simulink model "Modele_LQR_6DOF"  (R2024b)
settings: Solver=VariableStepAuto  StartTime=0.0  StopTime=50  FixedStep=0.0001  RelTol=1e-3
InitFcn:
  |     du0 = 0;
  |     du1 = 0;
  |     du2 = 0;
  |     du3 = 0;
  |     du4 = 0;
  |     du5 = 0;
  |     du6 = 0;
  |     du7 = 0;
values from neighbouring files (symbols this model uses):
  A_num = [0 0 0 0 0 0 0 0 0 0 0 0 ... (144 elements, 12x12)]    [Matrice_A_lineaire.mat]    (also in calcul_matrice_A_lineaire.m = double(A_num); resultats_stabilite.mat; testFinale.m = A_fcn(0, 0, 0, val_rll, val_ptc, val_yw, val_u, val_v, val_w; test_calcalV2.m = double(A_num))
  B = df_dcontrol    [Generate_PyMatrix.m]    (also in Parameters.m = -234.459; instabiliter_graphique.m = out.B_s.signals.values)
  Fx1 = -0.7071*force    (= -14.142)    [Parameters.m]
  Fx2 = -0.7071*force    (= -14.142)    [Parameters.m]
  Fx3 = 0    [Parameters.m]
  Fx4 = 0    [Parameters.m]
  Fx5 = 0    [Parameters.m]
  Fx6 = 0    [Parameters.m]
  Fx7 = 0.7071*force    (= 14.142)    [Parameters.m]
  Fx8 = 0.7071*force    (= 14.142)    [Parameters.m]
  Fy1 = 0.7071*force    (= 14.142)    [Parameters.m]
  Fy2 = -0.7071*force    (= -14.142)    [Parameters.m]
  Fy3 = 0    [Parameters.m]
  Fy4 = 0    [Parameters.m]
  Fy5 = 0    [Parameters.m]
  Fy6 = 0    [Parameters.m]
  Fy7 = 0.7071*force    (= 14.142)    [Parameters.m]
  Fy8 = -0.7071*force    (= -14.142)    [Parameters.m]
  Fz1 = 0    [Parameters.m]
  Fz2 = 0    [Parameters.m]
  Fz3 = -1*force    (= -20)    [Parameters.m]
  Fz4 = -1*force    (= -20)    [Parameters.m]
  Fz5 = -1*force    (= -20)    [Parameters.m]
  Fz6 = -1*force    (= -20)    [Parameters.m]
  Fz7 = 0    [Parameters.m]
  Fz8 = 0    [Parameters.m]
  I_x = 0.578    [Parameters.m]
  I_y = 0.645    [Parameters.m]
  I_z = 0.9366    [Parameters.m]
  lx1 = I_un_moteur(1)    [Calcul_Inertie_Nouveau.m]    (also in Parameters.m = 0.0194)
  lx2 = I_un_moteur(1)    [Calcul_Inertie_Nouveau.m]    (also in Parameters.m = 0.0194)
  lx3 = I_un_moteur(1)    [Calcul_Inertie_Nouveau.m]    (also in Parameters.m = -0.0317)
  lx4 = I_un_moteur(1)    [Calcul_Inertie_Nouveau.m]    (also in Parameters.m = -0.0317)
  lx5 = I_un_moteur(1)    [Calcul_Inertie_Nouveau.m]    (also in Parameters.m = 0.0317)
  lx6 = I_un_moteur(1)    [Calcul_Inertie_Nouveau.m]    (also in Parameters.m = 0.0317)
  lx7 = I_un_moteur(1)    [Calcul_Inertie_Nouveau.m]    (also in Parameters.m = -0.0194)
  lx8 = I_un_moteur(1)    [Calcul_Inertie_Nouveau.m]    (also in Parameters.m = -0.0194)
  ly1 = %.4f    [Calcul_Inertie_Nouveau.m]    (also in Parameters.m = 0.0381)
  ly2 = %.4f    [Calcul_Inertie_Nouveau.m]    (also in Parameters.m = -0.0381)
  ly3 = %.4f    [Calcul_Inertie_Nouveau.m]    (also in Parameters.m = 0.0049)
  ly4 = %.4f    [Calcul_Inertie_Nouveau.m]    (also in Parameters.m = -0.0049)
  ly5 = %.4f    [Calcul_Inertie_Nouveau.m]    (also in Parameters.m = 0.0049)
  ly6 = %.4f    [Calcul_Inertie_Nouveau.m]    (also in Parameters.m = -0.0049)
  ly7 = %.4f    [Calcul_Inertie_Nouveau.m]    (also in Parameters.m = 0.0381)
  ly8 = %.4f    [Calcul_Inertie_Nouveau.m]    (also in Parameters.m = -0.0381)
  lz1 = %.4f;\n', lx1, ly1, lz1)    [Calcul_Inertie_Nouveau.m]    (also in Parameters.m = 0.0575)
  lz2 = %.4f;\n', lx2, ly2, lz2)    [Calcul_Inertie_Nouveau.m]    (also in Parameters.m = 0.0575)
  lz3 = %.4f;\n', lx3, ly3, lz3)    [Calcul_Inertie_Nouveau.m]    (also in Parameters.m = 0.0366)
  lz4 = %.4f;\n', lx4, ly4, lz4)    [Calcul_Inertie_Nouveau.m]    (also in Parameters.m = 0.0366)
  lz5 = %.4f;\n', lx5, ly5, lz5)    [Calcul_Inertie_Nouveau.m]    (also in Parameters.m = 0.0366)
  lz6 = %.4f;\n', lx6, ly6, lz6)    [Calcul_Inertie_Nouveau.m]    (also in Parameters.m = 0.0366)
  lz7 = %.4f;\n', lx7, ly7, lz7)    [Calcul_Inertie_Nouveau.m]    (also in Parameters.m = 0.0575)
  lz8 = %.4f;\n', lx8, ly8, lz8)    [Calcul_Inertie_Nouveau.m]    (also in Parameters.m = 0.0575)
  m = 23.9    [Parameters.m]
  Q_envoyer = Q_final(:,:,1)    [Parameters.m]
  W = mass*gravity    (= 234.459)    [Generate_PyMatrix.m]    (also in Parameters.m; calcul_damping.m)
  x_rb = 0    [Parameters.m]
  x_rg = 0    [Parameters.m]
  y_rb = 0    [Parameters.m]
  y_rg = 0    [Parameters.m]
  z_rb = 0    [Parameters.m]
  z_rg = 0    [Parameters.m]
undefined symbols (not defined in the file or in its folder): sigbuilder_block
libraries: simulink x12, sharedtransform x1, dspinverses x1, SignalEditorBlockLib x1
(part 3 of 4)

== matlab function Modele_LQR_6DOF/Controller/MATLAB Function ==
  settings: updateMethod=DISCRETE
  data: R output; Q output; A output; B output; state input; Q_files input; Tau input; A_lineraire input

function [R,Q,A,B]= ABmatrix(state, Q_files, Tau, A_lineraire)
tic
    
    roll_ = state(4);
    pitch_ = state(5);
    yaw_ = state(6);
    u = state(7); %
    v = state(8); %
    w = state(9); %
    p = state(10);
    q = state(11);
    r = state(12);

    du0 = Tau(1);
    du1 = Tau(2);
    du2 = Tau(3);
    du3 = Tau(4);
    du4 = Tau(5);
    du5 = Tau(6);
    du6 = Tau(7);
    du7 = Tau(8);
    thrust = 0.1;
    importance = 0;

    % Q = Q_files;
    Q = diag([Q_files(1,1) Q_files(2,2) Q_files(3,3) Q_files(4,4) Q_files(5,5) Q_files(6,6) Q_files(7,7) Q_files(8,8) Q_files(9,9) Q_files(10,10) Q_files(11,11) Q_files(12,12)]);
    % Q = diag([80, 80, 80, 100, 100, 100, 50, 50, 50, 20, 20, 20]); % test répétition
    % Q = diag([4, 4, 4, 2, 2, 2, 1, 1, 1, 1, 1, 1]); % test ancien
    % R = diag([thrust, thrust, thrust-importance, thrust-importance, thrust-importance, thrust-importance, thrust, thrust]); 
    R = thrust*eye(8);

    radius = 0.26;
    
 % A = A_lineraire;

 % utiliser
%     A = [[0, 0, 0,   v*(sin(roll_)*sin(yaw_) + cos(roll_)*cos(yaw_)*sin(pitch_)) + w*(cos(roll_)*sin(yaw_) - cos(yaw_)*sin(pitch_)*sin(roll_)), w*cos(pitch_)*cos(roll_)*cos(yaw_) - u*cos(yaw_)*sin(pitch_) + v*cos(pitch_)*cos(yaw_)*sin(roll_), w*(cos(yaw_)*sin(roll_) - cos(roll_)*sin(pitch_)*sin(yaw_)) - v*(cos(roll_)*cos(yaw_) + sin(pitch_)*sin(roll_)*sin(yaw_)) - u*cos(pitch_)*sin(yaw_), cos(pitch_)*cos(yaw_), cos(yaw_)*sin(pitch_)*sin(roll_) - cos(roll_)*sin(yaw_), sin(roll_)*sin(yaw_) + cos(roll_)*cos(yaw_)*sin(pitch_),             0,                      0,                      0]
% [0, 0, 0, - v*(cos(yaw_)*sin(roll_) - cos(roll_)*sin(pitch_)*sin(yaw_)) - w*(cos(roll_)*cos(yaw_) + sin(pitch_)*sin(roll_)*sin(yaw_)), w*cos(pitch_)*cos(roll_)*sin(yaw_) - u*sin(pitch_)*sin(yaw_) + v*cos(pitch_)*sin(roll_)*sin(yaw_), w*(sin(roll_)*sin(yaw_) + cos(roll_)*cos(yaw_)*sin(pitch_)) - v*(cos(roll_)*sin(yaw_) - cos(yaw_)*sin(pitch_)*sin(roll_)) + u*cos(pitch_)*cos(yaw_), cos(pitch_)*sin(yaw_), cos(roll_)*cos(yaw_) + sin(pitch_)*sin(roll_)*sin(yaw_), cos(roll_)*sin(pitch_)*sin(yaw_) - cos(yaw_)*sin(roll_),             0,                      0,                      0]
% [0, 0, 0,                                                                         v*cos(pitch_)*cos(roll_) - w*cos(pitch_)*sin(roll_),                             - u*cos(pitch_) - w*cos(roll_)*sin(pitch_) - v*sin(pitch_)*sin(roll_),                                                                                                                                                   0,          -sin(pitch_),                                  cos(pitch_)*sin(roll_),                                  cos(pitch_)*cos(roll_),             0,                      0,                      0]
% [0, 0, 0,                                                                         q*cos(roll_)*tan(pitch_) - r*tan(pitch_)*sin(roll_),                               r*cos(roll_)*(tan(pitch_)^2 + 1) + q*sin(roll_)*(tan(pitch_)^2 + 1),                                                                                                                                                   0,                     0,                                                       0,                                                       0,             1, tan(pitch_)*sin(roll_), cos(roll_)*tan(pitch_)]
% [0, 0, 0,                                                                                               - r*cos(roll_) - q*sin(roll_),                                                                                                 0,                                                                                                                                                   0,                     0,                                                       0,                                                       0,             0,             cos(roll_),            -sin(roll_)]
% [0, 0, 0,                                                                     (q*cos(roll_))/cos(pitch_) - (r*sin(roll_))/cos(pitch_),               (r*cos(roll_)*sin(pitch_))/cos(pitch_)^2 + (q*sin(pitch_)*sin(roll_))/cos(pitch_)^2,                                                                                                                                                   0,                     0,                                                       0,                                                       0,             0, sin(roll_)/cos(pitch_), cos(roll_)/cos(pitch_)]
% [0, 0, 0,                                                                                                                           0,                                            (10*cos(pitch_)*(13080*pi*radius^3 - 234459/1000))/139,                                                                                                                                                   0,            -2221/1390,                                                       r,                                                      -q,             0,                     -w,                      v]
% [0, 0, 0,                                                          -(10*cos(pitch_)*cos(roll_)*(13080*pi*radius^3 - 234459/1000))/139,                                 (10*sin(pitch_)*sin(roll_)*(13080*pi*radius^3 - 234459/1000))/139,                                                                                                                                                   0,                    -r,                                               -1394/695,                                                       p,             w,                      0,                     -u]
% [0, 0, 0,                                                           (10*cos(pitch_)*sin(roll_)*(13080*pi*radius^3 - 234459/1000))/139,                                 (10*cos(roll_)*sin(pitch_)*(13080*pi*radius^3 - 234459/1000))/139,                                                                                                                                                   0,                     q,                                                      -p,                                               -2107/695,            -v,                      u,                      0]
% [0, 0, 0,                                                                                                                           0,                                                                                                 0,                                                                                                                                                   0,                     0,                                                       0,                                                       0, -193590/40171,           -(146*r)/289,           -(146*q)/289]
% [0, 0, 0,                                                                                                                           0,                                                                                                 0,                                                                                                                                                   0,                     0,                                                       0,                                                       0,   (359*r)/645,            -25812/5977,            (359*p)/645]
% [0, 0, 0,                                                                                                                           0,                                                                                                 0,                                                                                                                                                   0,                     0,                                                       0,                                                       0,   -(67*q)/937,            -(67*p)/937,         -387180/130243]];

% A displace wather 0.024

    A = [[0, 0, 0,   v*(sin(roll_)*sin(yaw_) + cos(roll_)*cos(yaw_)*sin(pitch_)) + w*(cos(roll_)*sin(yaw_) - cos(yaw_)*sin(pitch_)*sin(roll_)), w*cos(pitch_)*cos(roll_)*cos(yaw_) - u*cos(yaw_)*sin(pitch_) + v*cos(pitch_)*cos(yaw_)*sin(roll_), w*(cos(yaw_)*sin(roll_) - cos(roll_)*sin(pitch_)*sin(yaw_)) - v*(cos(roll_)*cos(yaw_) + sin(pitch_)*sin(roll_)*sin(yaw_)) - u*cos(pitch_)*sin(yaw_),                           cos(pitch_)*cos(yaw_), cos(yaw_)*sin(pitch_)*sin(roll_) - cos(roll_)*sin(yaw_), sin(roll_)*sin(yaw_) + cos(roll_)*cos(yaw_)*sin(pitch_),                                             0,                                             0,                                             0]
[0, 0, 0, - v*(cos(yaw_)*sin(roll_) - cos(roll_)*sin(pitch_)*sin(yaw_)) - w*(cos(roll_)*cos(yaw_) + sin(pitch_)*sin(roll_)*sin(yaw_)), w*cos(pitch_)*cos(roll_)*sin(yaw_) - u*sin(pitch_)*sin(yaw_) + v*cos(pitch_)*sin(roll_)*sin(yaw_), w*(sin(roll_)*sin(yaw_) + cos(roll_)*cos(yaw_)*sin(pitch_)) - v*(cos(roll_)*sin(yaw_) - cos(yaw_)*sin(pitch_)*sin(roll_)) + u*cos(pitch_)*cos(yaw_),                           cos(pitch_)*sin(yaw_), cos(roll_)*cos(yaw_) + sin(pitch_)*sin(roll_)*sin(yaw_), cos(roll_)*sin(pitch_)*sin(yaw_) - cos(yaw_)*sin(roll_),                                             0,                                             0,                                             0]
[0, 0, 0,                                                                         v*cos(pitch_)*cos(roll_) - w*cos(pitch_)*sin(roll_),                             - u*cos(pitch_) - w*cos(roll_)*sin(pitch_) - v*sin(pitch_)*sin(roll_),                                                                                                                                                   0,                                    -sin(pitch_),                                  cos(pitch_)*sin(roll_),                                  cos(pitch_)*cos(roll_),                                             0,                                             0,                                             0]
[0, 0, 0,                                                                         q*cos(roll_)*tan(pitch_) - r*tan(pitch_)*sin(roll_),                               r*cos(roll_)*(tan(pitch_)^2 + 1) + q*sin(roll_)*(tan(pitch_)^2 + 1),                                                                                                                                                   0,                                               0,                                                       0,                                                       0,                                             1,                        tan(pitch_)*sin(roll_),                        cos(roll_)*tan(pitch_)]
[0, 0, 0,                                                                                               - r*cos(roll_) - q*sin(roll_),                                                                                                 0,                                                                                                                                                   0,                                               0,                                                       0,                                                       0,                                             0,                                    cos(roll_),                                   -sin(roll_)]
[0, 0, 0,                                                                     (q*cos(roll_))/cos(pitch_) - (r*sin(roll_))/cos(pitch_),               (r*cos(roll_)*sin(pitch_))/cos(pitch_)^2 + (q*sin(pitch_)*sin(roll_))/cos(pitch_)^2,                                                                                                                                                   0,                                               0,                                                       0,                                                       0,                                             0,                        sin(roll_)/cos(pitch_),                        cos(roll_)/cos(pitch_)]
[0, 0, 0,                                                                                                                           0,                                               (34515869019144192*cos(pitch_))/1177950653953795175,                                                                                                                                                   0,        -1781159578876195687/1177950653953795175,                 (52306257075229432*r)/47118026158151807,                -(52306257075229432*q)/47118026158151807,                                             0,      -(52306257075229432*w)/47118026158151807,       (52306257075229432*v)/47118026158151807]
[0, 0, 0,                                                               -(4314483627393024*cos(pitch_)*cos(roll_))/163457053360091975,                                      (4314483627393024*sin(pitch_)*sin(roll_))/163457053360091975,                                                                                                                                                   0,        -(47118026158151807*r)/52306257075229432,                     -21772599621964530/6538282134403679,                                                       p,                                             w,                                             0,      -(47118026158151807*u)/52306257075229432]
[0, 0, 0,                                                                (4314483627393024*cos(pitch_)*sin(roll_))/163457053360091975,                                      (4314483627393024*cos(roll_)*sin(pitch_))/163457053360091975,                                                                                                                                                   0,         (47118026158151807*q)/52306257075229432,                                                      -p,                     -30037936391212500/6538282134403679,                                            -v,       (47118026158151807*u)/52306257075229432,                                             0]
[0, 0, 0,                                                                                          -(5886*cos(pitch_)*cos(roll_))/289,                                                                 (5886*sin(pitch_)*sin(roll_))/289,                                                                                                                                                   0,                                               0,                                                       0,                                                       0,                                   -21001/2890, -(4529701451644209453*r)/10412322338480586752, -(4529701451644209453*q)/10412322338480586752]
[0, 0, 0,                                                                                                                           0,                                         -(424130998507243831296*cos(pitch_))/23969076990356289235,                                                                                                                                                   0,    (26563742295437440000*w)/4793815398071257847,                                                       0,            (26563742295437440000*u)/4793815398071257847, (12203835216683534637*r)/23969076990356289235, -1173259760524052135936/119845384951781446175, (12203835216683534637*p)/23969076990356289235]
[0, 0, 0,                                                                                                                           0,                                                                                                 0,                                                                                                                                                   0, -(132818711477187200000*v)/33028479893644708141,         -(132818711477187200000*u)/33028479893644708141,                                                       0, -(3144432313395115731*q)/33028479893644708141, -(3144432313395115731*p)/33028479893644708141,     -33128478858937368576/7180104324705371335]];
    
    % original
    A = [[ 0, 0, 0,   v*(sin(roll_)*sin(yaw_) + cos(roll_)*cos(yaw_)*sin(pitch_)) + w*(cos(roll_)*sin(yaw_) - cos(yaw_)*sin(pitch_)*sin(roll_)), w*cos(pitch_)*cos(roll_)*cos(yaw_) - u*cos(yaw_)*sin(pitch_) + v*cos(pitch_)*cos(yaw_)*sin(roll_), w*(cos(yaw_)*sin(roll_) - cos(roll_)*sin(pitch_)*sin(yaw_)) - v*(cos(roll_)*cos(yaw_) + sin(pitch_)*sin(roll_)*sin(yaw_)) - u*cos(pitch_)*sin(yaw_), cos(pitch_)*cos(yaw_), cos(yaw_)*sin(pitch_)*sin(roll_) - cos(roll_)*sin(yaw_), sin(roll_)*sin(yaw_) + cos(roll_)*cos(yaw_)*sin(pitch_),          0,                      0,                      0]
[ 0, 0, 0, - v*(cos(yaw_)*sin(roll_) - cos(roll_)*sin(pitch_)*sin(yaw_)) - w*(cos(roll_)*cos(yaw_) + sin(pitch_)*sin(roll_)*sin(yaw_)), w*cos(pitch_)*cos(roll_)*sin(yaw_) - u*sin(pitch_)*sin(yaw_) + v*cos(pitch_)*sin(roll_)*sin(yaw_), w*(sin(roll_)*sin(yaw_) + cos(roll_)*cos(yaw_)*sin(pitch_)) - v*(cos(roll_)*sin(yaw_) - cos(yaw_)*sin(pitch_)*sin(roll_)) + u*cos(pitch_)*cos(yaw_), cos(pitch_)*sin(yaw_), cos(roll_)*cos(yaw_) + sin(pitch_)*sin(roll_)*sin(yaw_), cos(roll_)*sin(pitch_)*sin(yaw_) - cos(yaw_)*sin(roll_),          0,                      0,                      0]
[ 0, 0, 0,                                                                         v*cos(pitch_)*cos(roll_) - w*cos(pitch_)*sin(roll_),                             - u*cos(pitch_) - w*cos(roll_)*sin(pitch_) - v*sin(pitch_)*sin(roll_),                                                                                                                                                   0,          -sin(pitch_),                                  cos(pitch_)*sin(roll_),                                  cos(pitch_)*cos(roll_),          0,                      0,                      0]
[ 0, 0, 0,                                                                         q*cos(roll_)*tan(pitch_) - r*tan(pitch_)*sin(roll_),                               r*cos(roll_)*(tan(pitch_)^2 + 1) + q*sin(roll_)*(tan(pitch_)^2 + 1),                                                                                                                                                   0,                     0,                                                       0,                                                       0,          1, tan(pitch_)*sin(roll_), cos(roll_)*tan(pitch_)]
[ 0, 0, 0,                                                                                               - r*cos(roll_) - q*sin(roll_),                                                                                                 0,                                                                                                                                                   0,                     0,                                                       0,                                                       0,          0,             cos(roll_),            -sin(roll_)]
[ 0, 0, 0,                                                                     (q*cos(roll_))/cos(pitch_) - (r*sin(roll_))/cos(pitch_),               (r*cos(roll_)*sin(pitch_))/cos(pitch_)^2 + (q*sin(pitch_)*sin(roll_))/cos(pitch_)^2,                                                                                                                                                   0,                     0,                                                       0,                                                       0,          0, sin(roll_)/cos(pitch_), cos(roll_)/cos(pitch_)]
[ 0, 0, 0,                                                                                                                           0,                                                    (7873445366256113*cos(pitch_))/395824185999360,                                                                                                                                                   0,             2221/2250,                                               (17*r)/25,                                          -(1343*q)/2250,          0,         -(1343*w)/2250,              (17*v)/25]
[ 0, 0, 0,                                                                   -(2315719225369445*cos(pitch_)*cos(roll_))/79164837199872,                                          (2315719225369445*sin(pitch_)*sin(roll_))/79164837199872,                                                                                                                                                   0,            -(25*r)/17,                                                   82/45,                                               (79*p)/90,  (79*w)/90,                      0,             -(25*u)/17]
[ 0, 0, 0,                                                                      (146564507934775*cos(pitch_)*sin(roll_))/4398046511104,                                            (146564507934775*cos(roll_)*sin(pitch_))/4398046511104,                                                                                                                                                   0,         (2250*q)/1343,                                              -(90*p)/79,                                               4214/1343, -(90*v)/79,          (2250*u)/1343,                      0]
[ 0, 0, 0,                                                                                                                           0,                                                                                                 0,                                                                                                                                                   0,                     0,                                               (187*w)/4,                                               (187*v)/4,       81/2,                      0,                      0]
[ 0, 0, 0,                                                                                                                           0,                                                                                                 0,                                                                                                                                                   0,            -(907*w)/4,                                                       0,                                              -(907*u)/4,          0,                   81/2,                      0]
[ 0, 0, 0,                                                                                                                           0,                                                                                                 0,                                                                                                                                                   0,                 180*v,                                                   180*u,                                                       0,          0,                      0,                   81/2]];

% utiliser
%     B = [[                                          0,                                            0,              0,              0,             0,             0,                                            0,                                           0]
% [                                          0,                                            0,              0,              0,             0,             0,                                            0,                                           0]
% [                                          0,                                            0,              0,              0,             0,             0,                                            0,                                           0]
% [                                          0,                                            0,              0,              0,             0,             0,                                            0,                                           0]
% [                                          0,                                            0,              0,              0,             0,             0,                                            0,                                           0]
% [                                          0,                                            0,              0,              0,             0,             0,                                            0,                                           0]
% [                                  -707/6950,                                    -707/6950,              0,              0,             0,             0,                                     707/6950,                                    707/6950]
% [                                   707/6950,                                    -707/6950,              0,              0,             0,             0,                                     707/6950,                                   -707/6950]
% [                                          0,                                            0,        -20/139,        -20/139,       -20/139,       -20/139,                                            0,                                           0]
% [                                          0,                                            0,  -130255/80342,   130255/80342, -130255/80342,  130255/80342,                                            0,                                           0]
% [                                          0,                                            0, -256447/448275, -256447/448275, 256447/448275, 256447/448275,                                            0,                                           0]
% [194698457386957391875/146640581566903877632, -194698457386957391875/146640581566903877632,              0,              0,             0,             0, -194698457386957391875/146640581566903877632, 194698457386957391875/146640581566903877632]];

% matrice B displace wather 0.024

    B = [[                                        0,                                          0,                                           0,                                           0,                                          0,                                          0,                                          0,                                         0]
[                                        0,                                          0,                                           0,                                           0,                                          0,                                          0,                                          0,                                         0]
[                                        0,                                          0,                                           0,                                           0,                                          0,                                          0,                                          0,                                         0]
[                                        0,                                          0,                                           0,                                           0,                                          0,                                          0,                                          0,                                         0]
[                                        0,                                          0,                                           0,                                           0,                                          0,                                          0,                                          0,                                         0]
[                                        0,                                          0,                                           0,                                           0,                                          0,                                          0,                                          0,                                         0]
[   -24875351066804224/1177950653953795175,     -24875351066804224/1177950653953795175,                                           0,                                           0,                                          0,                                          0,      24875351066804224/1177950653953795175,     24875351066804224/1177950653953795175]
[      3109418883350528/163457053360091975,       -3109418883350528/163457053360091975,                                           0,                                           0,                                          0,                                          0,        3109418883350528/163457053360091975,      -3109418883350528/163457053360091975]
[                                        0,                                          0,           -175921860444160/6538282134403679,           -175921860444160/6538282134403679,          -175921860444160/6538282134403679,          -175921860444160/6538282134403679,                                          0,                                         0]
[                                        0,                                          0,                                   -545/1156,                                    545/1156,                                  -545/1156,                                   545/1156,                                          0,                                         0]
[                                        0,                                          0, -19329449600674168832/119845384951781446175, -19329449600674168832/119845384951781446175, 19329449600674168832/119845384951781446175, 19329449600674168832/119845384951781446175,                                          0,                                         0]
[13034206352264930000/33028479893644708141, -13034206352264930000/33028479893644708141,                                           0,                                           0,                                          0,                                          0, -13034206352264930000/33028479893644708141, 13034206352264930000/33028479893644708141]]; 

% 
% B = [[                                                                                                                                              0,                                                                                                                                                 0,                                                                                                                                                   0,                                                                                                                                                   0,                                                                                                                                                 0,                                                                                                                                                 0,                                                                                                                                                 0,                                                                                                                                               0]
% [                                                                                                                                              0,                                                                                                                                                 0,                                                                                                                                                   0,                                                                                                                                                   0,                                                                                                                                                 0,                                                                                                                                                 0,                                                                                                                                                 0,                                                                                                                                               0]
% [                                                                                                                                              0,                                                                                                                                                 0,                                                                                                                                                   0,                                                                                                                                                   0,                                                                                                                                                 0,                                                                                                                                                 0,                                                                                                                                                 0,                                                                                                                                               0]
% [                                                                                                                                              0,                                                                                                                                                 0,                                                                                                                                                   0,                                                                                                                                                   0,                                                                                                                                                 0,                                                                                                                                                 0,                                                                                                                                                 0,                                                                                                                                               0]
% [                                                                                                                                              0,                                                                                                                                                 0,                                                                                                                                                   0,                                                                                                                                                   0,                                                                                                                                                 0,                                                                                                                                                 0,                                                                                                                                                 0,                                                                                                                                               0]
% [                                                                                                                                              0,                                                                                                                                                 0,                                                                                                                                                   0,                                                                                                                                                   0,                                                                                                                                                 0,                                                                                                                                                 0,                                                                                                                                                 0,                                                                                                                                               0]
% [     - (24875351066804224*abs(du0))/1177950653953795175 - (12437675533402112*du0*(du0 + conj(du0)))/(1177950653953795175*(du0*conj(du0))^(1/2)),        - (24875351066804224*abs(du1))/1177950653953795175 - (12437675533402112*du1*(du1 + conj(du1)))/(1177950653953795175*(du1*conj(du1))^(1/2)),                                                                                                                                                   0,                                                                                                                                                   0,                                                                                                                                                 0,                                                                                                                                                 0,          (24875351066804224*abs(du6))/1177950653953795175 + (12437675533402112*du6*(du6 + conj(du6)))/(1177950653953795175*(du6*conj(du6))^(1/2)),        (24875351066804224*abs(du7))/1177950653953795175 + (12437675533402112*du7*(du7 + conj(du7)))/(1177950653953795175*(du7*conj(du7))^(1/2))]
% [           (3109418883350528*abs(du0))/163457053360091975 + (1554709441675264*du0*(du0 + conj(du0)))/(163457053360091975*(du0*conj(du0))^(1/2)),            - (3109418883350528*abs(du1))/163457053360091975 - (1554709441675264*du1*(du1 + conj(du1)))/(163457053360091975*(du1*conj(du1))^(1/2)),                                                                                                                                                   0,                                                                                                                                                   0,                                                                                                                                                 0,                                                                                                                                                 0,              (3109418883350528*abs(du6))/163457053360091975 + (1554709441675264*du6*(du6 + conj(du6)))/(163457053360091975*(du6*conj(du6))^(1/2)),          - (3109418883350528*abs(du7))/163457053360091975 - (1554709441675264*du7*(du7 + conj(du7)))/(163457053360091975*(du7*conj(du7))^(1/2))]
% [                                                                                                                                              0,                                                                                                                                                 0,                     - (175921860444160*abs(du2))/6538282134403679 - (87960930222080*du2*(du2 + conj(du2)))/(6538282134403679*(du2*conj(du2))^(1/2)),                     - (175921860444160*abs(du3))/6538282134403679 - (87960930222080*du3*(du3 + conj(du3)))/(6538282134403679*(du3*conj(du3))^(1/2)),                   - (175921860444160*abs(du4))/6538282134403679 - (87960930222080*du4*(du4 + conj(du4)))/(6538282134403679*(du4*conj(du4))^(1/2)),                   - (175921860444160*abs(du5))/6538282134403679 - (87960930222080*du5*(du5 + conj(du5)))/(6538282134403679*(du5*conj(du5))^(1/2)),                                                                                                                                                 0,                                                                                                                                               0]
% [                                                                                                                                              0,                                                                                                                                                 0,                                                                    - (545*abs(du2))/1156 - (545*du2*(du2 + conj(du2)))/(2312*(du2*conj(du2))^(1/2)),                                                                      (545*abs(du3))/1156 + (545*du3*(du3 + conj(du3)))/(2312*(du3*conj(du3))^(1/2)),                                                                  - (545*abs(du4))/1156 - (545*du4*(du4 + conj(du4)))/(2312*(du4*conj(du4))^(1/2)),                                                                    (545*abs(du5))/1156 + (545*du5*(du5 + conj(du5)))/(2312*(du5*conj(du5))^(1/2)),                                                                                                                                                 0,                                                                                                                                               0]
% [                                                                                                                                              0,                                                                                                                                                 0, - (19329449600674168832*abs(du2))/119845384951781446175 - (9664724800337084416*du2*(du2 + conj(du2)))/(119845384951781446175*(du2*conj(du2))^(1/2)), - (19329449600674168832*abs(du3))/119845384951781446175 - (9664724800337084416*du3*(du3 + conj(du3)))/(119845384951781446175*(du3*conj(du3))^(1/2)), (19329449600674168832*abs(du4))/119845384951781446175 + (9664724800337084416*du4*(du4 + conj(du4)))/(119845384951781446175*(du4*conj(du4))^(1/2)), (19329449600674168832*abs(du5))/119845384951781446175 + (9664724800337084416*du5*(du5 + conj(du5)))/(119845384951781446175*(du5*conj(du5))^(1/2)),                                                                                                                                                 0,                                                                                                                                               0]
% [(13034206352264930000*abs(du0))/33028479893644708141 + (6517103176132465000*du0*(du0 + conj(du0)))/(33028479893644708141*(du0*conj(du0))^(1/2)), - (13034206352264930000*abs(du1))/33028479893644708141 - (6517103176132465000*du1*(du1 + conj(du1)))/(33028479893644708141*(du1*conj(du1))^(1/2)),                                                                                                                                                   0,                                                                                                                                                   0,                                                                                                                                                 0,                                                                                                                                                 0, - (13034206352264930000*abs(du6))/33028479893644708141 - (6517103176132465000*du6*(du6 + conj(du6)))/(33028479893644708141*(du6*conj(du6))^(1/2)), (13034206352264930000*abs(du7))/33028479893644708141 + (6517103176132465000*du7*(du7 + conj(du7)))/(33028479893644708141*(du7*conj(du7))^(1/2))]]; 

% matrice original
%     B = [[                                   0,                                    0,         0,         0,         0,         0,                                    0,                                   0]
% [                                   0,                                    0,         0,         0,         0,         0,                                    0,                                   0]
% [                                   0,                                    0,         0,         0,         0,         0,                                    0,                                   0]
% [                                   0,                                    0,         0,         0,         0,         0,                                    0,                                   0]
% [                                   0,                                    0,         0,         0,         0,         0,                                    0,                                   0]
% [                                   0,                                    0,         0,         0,         0,         0,                                    0,                                   0]
% [                          -707/11250,                           -707/11250,         0,         0,         0,         0,                            707/11250,                           707/11250]
% [                            707/7650,                            -707/7650,         0,         0,         0,         0,                             707/7650,                           -707/7650]
% [                                   0,                                    0, -200/1343, -200/1343, -200/1343, -200/1343,                                    0,                                   0]
% [                                   0,                                    0,    -109/8,     109/8,    -109/8,     109/8,                                    0,                                   0]
% [                                   0,                                    0, -1073/200, -1073/200,  1073/200,  1073/200,                                    0,                                   0]
% [ 162927579403311625/9007199254740992, -162927579403311625/9007199254740992,         0,         0,         0,         0, -162927579403311625/9007199254740992, 162927579403311625/9007199254740992]];

toc
end
